simulink model "exp4_nonmin"  (R2024b)
settings: Solver=ode45  StartTime=0.0  StopTime=15  MaxStep=0.01  RelTol=1e-3
settings Model: Creator=1  LastModifiedBy=1

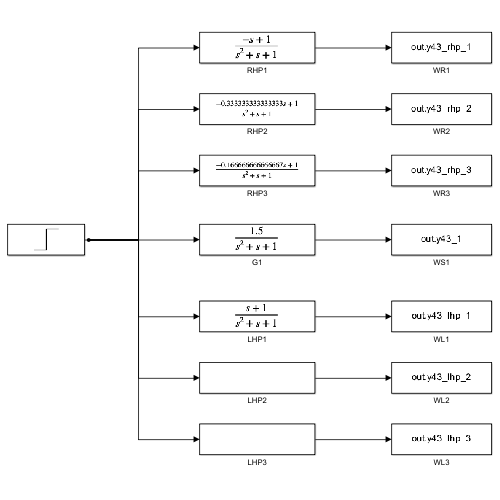
[thumbnail: Simulink's stored preview of the top-level diagram]
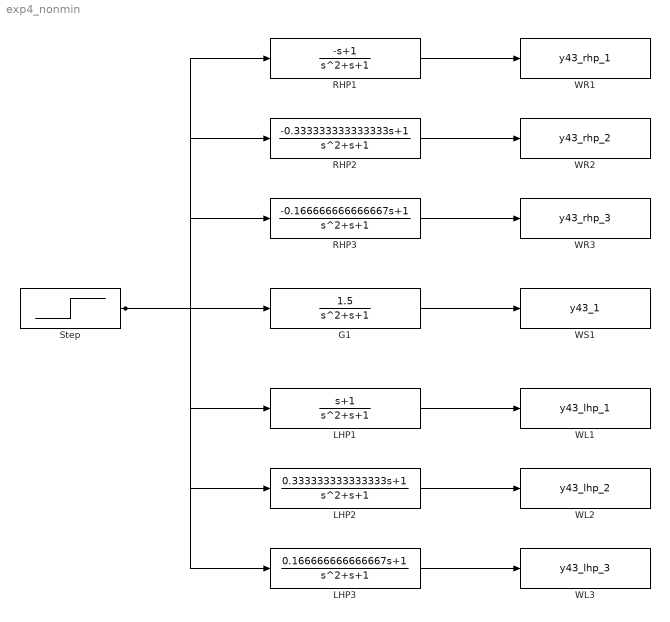
== system exp4_nonmin ==
  G1 : TransferFcn  Numerator=[1.5]  Denominator=[1 1 1]
  LHP1 : TransferFcn  Numerator=[1 1]  Denominator=[1 1 1]
  LHP2 : TransferFcn  Numerator=[0.333333333333333 1]  Denominator=[1 1 1]
  LHP3 : TransferFcn  Numerator=[0.166666666666667 1]  Denominator=[1 1 1]
  RHP1 : TransferFcn  Numerator=[-1 1]  Denominator=[1 1 1]
  RHP2 : TransferFcn  Numerator=[-0.333333333333333 1]  Denominator=[1 1 1]
  RHP3 : TransferFcn  Numerator=[-0.166666666666667 1]  Denominator=[1 1 1]
  Step : Step  Time=0  SampleTime=0
  WL1 : ToWorkspace  VariableName=y43_lhp_1  SaveFormat=Timeseries  SampleTime=-1
  WL2 : ToWorkspace  VariableName=y43_lhp_2  SaveFormat=Timeseries  SampleTime=-1
  WL3 : ToWorkspace  VariableName=y43_lhp_3  SaveFormat=Timeseries  SampleTime=-1
  WR1 : ToWorkspace  VariableName=y43_rhp_1  SaveFormat=Timeseries  SampleTime=-1
  WR2 : ToWorkspace  VariableName=y43_rhp_2  SaveFormat=Timeseries  SampleTime=-1
  WR3 : ToWorkspace  VariableName=y43_rhp_3  SaveFormat=Timeseries  SampleTime=-1
  WS1 : ToWorkspace  VariableName=y43_1  SaveFormat=Timeseries  SampleTime=-1
  wires:
  Step/1 -> G1/1, RHP1/1, RHP2/1, RHP3/1, LHP1/1, LHP2/1, LHP3/1
  G1/1 -> WS1/1
  RHP1/1 -> WR1/1
  RHP2/1 -> WR2/1
  RHP3/1 -> WR3/1
  LHP1/1 -> WL1/1
  LHP2/1 -> WL2/1
  LHP3/1 -> WL3/1
